simulink model "slip_angle"  (R2015a)
settings: Solver=ode3  StartTime=0  StopTime=5  RelTol=1e-3
settings Model: Creator=BML  LastModifiedBy=BML
settings SolverCC: AutoInsertRateTranBlk=on

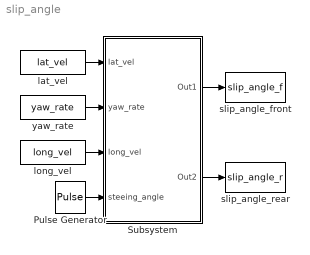
== system slip_angle ==
  Pulse Generator : DiscretePulseGenerator  Amplitude=0  Period=10  PulseWidth=10
  Subsystem : Subsystem
  lat_vel : FromWorkspace  VariableName=lat_vel  SampleTime=0
  long_vel : FromWorkspace  VariableName=long_vel  SampleTime=0
  slip_angle_front : ToWorkspace  VariableName=slip_angle_f  SaveFormat=Timeseries  SampleTime=-1
  slip_angle_rear : ToWorkspace  VariableName=slip_angle_r  SaveFormat=Timeseries  SampleTime=-1
  yaw_rate : FromWorkspace  VariableName=yaw_rate  SampleTime=0
  wires:
  lat_vel/1 -> Subsystem/1(lat_vel)
  yaw_rate/1 -> Subsystem/2(yaw_rate)
  long_vel/1 -> Subsystem/3(long_vel)
  Pulse Generator/1 -> Subsystem/4("steeing_angle ")
  Subsystem/1(Out1) -> slip_angle_front/1
  Subsystem/2(Out2) -> slip_angle_rear/1

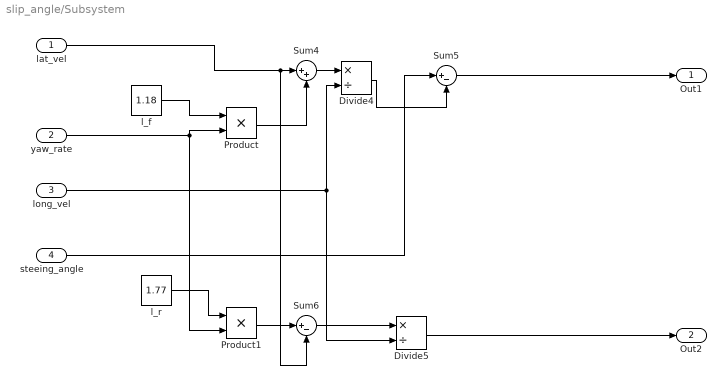
== system slip_angle/Subsystem ==
  lat_vel : Inport
  yaw_rate : Inport  Port=2
  long_vel : Inport  Port=3
  "steeing_angle " : Inport  Port=4
  Divide4 : Product  Inputs=*/
  Divide5 : Product  Inputs=*/
  Product : Product
  Product1 : Product
  Sum4 : Sum  Inputs=|++
  Sum5 : Sum  Inputs=|+-
  Sum6 : Sum  Inputs=|+-
  l_f : Constant  Value=1.18
  l_r : Constant  Value=1.77
  Out1 : Outport
  Out2 : Outport  Port=2
  wires:
  yaw_rate/1 -> Product1/2, Product/2
  long_vel/1 -> Divide5/2, Divide4/2
  l_f/1 -> Product/1
  lat_vel/1 -> Sum6/2, Sum4/1
  Divide4/1 -> Sum5/2
  Product/1 -> Sum4/2
  Sum4/1 -> Divide4/1
  Divide5/1 -> Out2/1
  "steeing_angle "/1 -> Sum5/1
  Sum5/1 -> Out1/1
  Product1/1 -> Sum6/1
  l_r/1 -> Product1/1
  Sum6/1 -> Divide5/1
